simulink model "current_position_feedback"  (R2023b)
settings: Solver=VariableStepAuto  StartTime=0.0  StopTime=4  RelTol=1e-3
values from neighbouring files (symbols this model uses):
  p_controller = p_controller.C    [MotorControlPosition.m]
  plant = 1/s*( (El*Me) / (1+(El*Me*Kt)) )    [MotorControlPosition.m]
libraries: cstblocks x3, simulink x1
settings Model: PacingRate=0.710000  Creator=frenci  LastModifiedBy=frenci

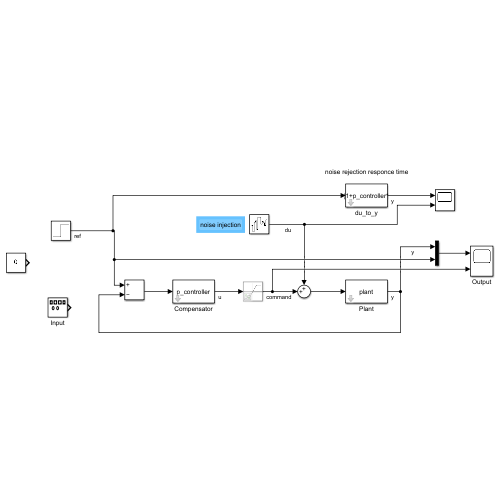
[thumbnail: Simulink's stored preview of the top-level diagram]
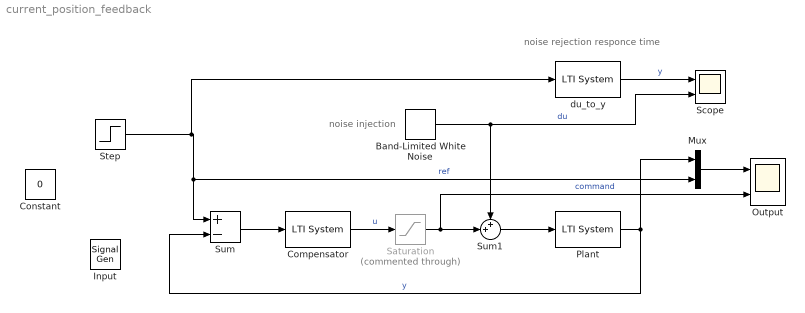
== system current_position_feedback ==
  note: noise rejection responce time
  note: noise injection
  Band-Limited White Noise : simulink/Sources/Band-Limited White Noise  Cov=[0.1]  Ts=0.8  seed=[23341]
  Compensator : cstblocks/LTI System  sys=p_controller  IC=[]  PadeOrder=0
  Constant : Constant  Value=0
  Input : SignalGenerator
  Mux : Mux  Inputs=2
  Output : Scope  NumInputPorts=2
  Plant : cstblocks/LTI System  sys=plant  IC=[]  PadeOrder=0
  Saturation : Saturate  Commented=through  UpperLimit=100  LowerLimit=-100
  Scope : Scope  NumInputPorts=2
  Step : Step  SampleTime=0
  Sum : Sum  Inputs=+-
  Sum1 : Sum  Inputs=++|
  du_to_y : cstblocks/LTI System  sys=plant/(1+p_controller*plant)  IC=[]  PadeOrder=0
  wires:
  Sum/1 -> Compensator/1
  Compensator/1 -> Saturation/1  "u"
  Plant/1 -> Sum/2, Mux/1  "y"
  Mux/1 -> Output/1
  du_to_y/1 -> Scope/1  "y"
  Step/1 -> du_to_y/1, Sum/1, Mux/2  "ref"
  Saturation/1 -> Output/2, Sum1/2  "command"
  Sum1/1 -> Plant/1
  Band-Limited White Noise/1 -> Scope/2, Sum1/1  "du"
